simulink model "W3P3"  (R2020b)
settings: Solver=VariableStepAuto  StartTime=0.0  StopTime=10.0  RelTol=1e-3
undefined symbols (not defined in the file or in its folder): DOWN_TABLE, DOWN_TH_BP, EMAP, Iei, Kfactor, NE_VEC, speedratio, TH_VEC, Torkratio, UP_TABLE, UP_TH_BP
settings Model: Creator=saadh  LastModifiedBy=saadh

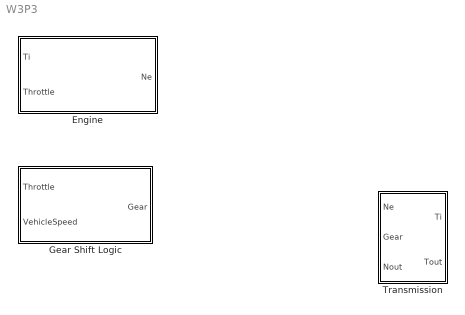
== system W3P3 ==
  Engine : Subsystem
  Gear Shift Logic : Stateflow chart  TreatAsAtomicUnit=on
  Transmission : Subsystem

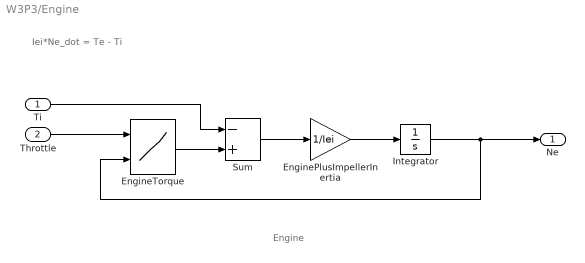
== system W3P3/Engine ==
  note: Engine
  note: Iei*Ne_dot = Te - Ti
  Ti : Inport  Unit=ft*lbf@torque
  Throttle : Inport  Port=2  Unit=%
  EnginePlusImpellerInertia : Gain  Gain=1/Iei  SaturateOnIntegerOverflow=on  OutDataTypeStr=Inherit: Same as input  ParamDataTypeStr=Inherit: Same as input
  EngineTorque : Lookup_n-D  BreakpointsForDimension1=TH_VEC  BreakpointsForDimension2=NE_VEC  Table=EMAP  InputSameDT=on
      settings: InputPortMap=u0,u1
  Integrator : Integrator  InitialCondition=1000  LimitOutput=on  UpperSaturationLimit=6000  LowerSaturationLimit=600  ZeroCross=off
  Sum : Sum  Inputs=-+  InputSameDT=on  SaturateOnIntegerOverflow=on  OutDataTypeStr=Inherit: Same as first input
  Ne : Outport  Unit=rpm  VectorParamsAs1DForOutWhenUnconnected=off
  wires:
  EngineTorque/1 -> Sum/2
  EnginePlusImpellerInertia/1 -> Integrator/1
  Integrator/1 -> Ne/1, EngineTorque/2
  Sum/1 -> EnginePlusImpellerInertia/1
  Throttle/1 -> EngineTorque/1
  Ti/1 -> Sum/1

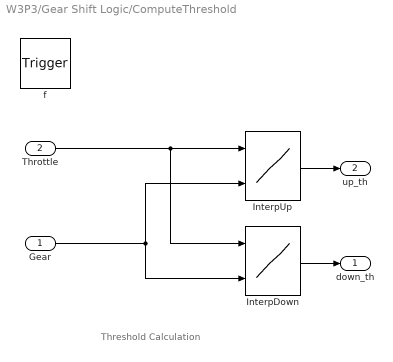
== system W3P3/Gear Shift Logic/ComputeThreshold ==
  note: Threshold Calculation
  Gear : Inport
  Throttle : Inport  Port=2
  f : TriggerPort  TriggerType=function-call  VariantControl=(inherit)
      settings: CopyFcn=Stateflow.SLINSF.SimulinkMan.removeBlockPreDeleteFcn  PreDeleteFcn=Stateflow.SLINSF.SimulinkMan.unsafePredeleteFcn
  InterpDown : Lookup_n-D  BreakpointsForDimension1=DOWN_TH_BP  BreakpointsForDimension2=[1:4]  Table=DOWN_TABLE  OutDataTypeStr=double  LockScale=on
      settings: InputPortMap=u0,u1
  InterpUp : Lookup_n-D  BreakpointsForDimension1=UP_TH_BP  BreakpointsForDimension2=[1:4]  Table=UP_TABLE  OutDataTypeStr=double  LockScale=on
      settings: InputPortMap=u0,u1
  down_th : Outport  InitialOutput=0  VectorParamsAs1DForOutWhenUnconnected=off
  up_th : Outport  Port=2  InitialOutput=0  VectorParamsAs1DForOutWhenUnconnected=off
  wires:
  Gear/1 -> InterpDown/2, InterpUp/2
  InterpUp/1 -> up_th/1
  Throttle/1 -> InterpDown/1, InterpUp/1
  InterpDown/1 -> down_th/1

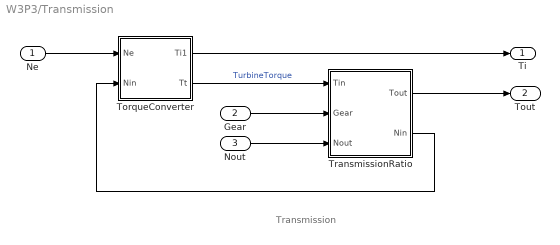
== system W3P3/Transmission ==
  note: Transmission
  Ne : Inport
  Gear : Inport  Port=2  Unit=1
  Nout : Inport  Port=3  Unit=rpm
  TorqueConverter : Subsystem
  TransmissionRatio : Subsystem
  Ti : Outport  VectorParamsAs1DForOutWhenUnconnected=off
  Tout : Outport  Port=2  Unit=ft*lbf@torque  VectorParamsAs1DForOutWhenUnconnected=off
  wires:
  Ne/1 -> TorqueConverter/1(Ne)
  TorqueConverter/2(Tt) -> TransmissionRatio/1(Tin)  "TurbineTorque"
  TransmissionRatio/1(Tout) -> Tout/1
  Gear/1 -> TransmissionRatio/2(Gear)
  TransmissionRatio/2(Nin) -> TorqueConverter/2(Nin)
  TorqueConverter/1(Ti1) -> Ti/1
  Nout/1 -> TransmissionRatio/3(Nout)

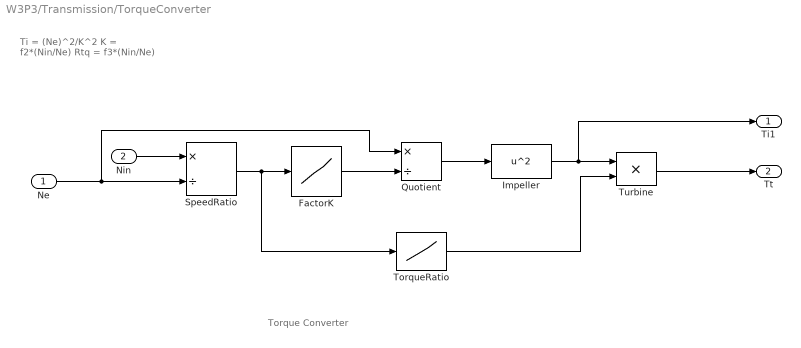
== system W3P3/Transmission/TorqueConverter ==
  note: Ti = (Ne)^2/K^2
      | K = f2*(Nin/Ne)
      | Rtq = f3*(Nin/Ne)
  note: Torque Converter
  Ne : Inport
  Nin : Inport  Port=2
  FactorK : Lookup_n-D  NumberOfTableDimensions=1  BreakpointsForDimension1=speedratio  Table=Kfactor  SaturateOnIntegerOverflow=on  InputSameDT=on
  Impeller : Fcn  Expr=u^2
  Quotient : Product  Inputs=*/  InputSameDT=on  SaturateOnIntegerOverflow=on  OutDataTypeStr=Inherit: Same as first input
  SpeedRatio : Product  Inputs=*/  InputSameDT=on  SaturateOnIntegerOverflow=on  OutDataTypeStr=Inherit: Same as first input
  TorqueRatio : Lookup_n-D  NumberOfTableDimensions=1  BreakpointsForDimension1=speedratio  Table=Torkratio  SaturateOnIntegerOverflow=on  InputSameDT=on
  Turbine : Product  InputSameDT=on  SaturateOnIntegerOverflow=on  OutDataTypeStr=Inherit: Same as first input
  Ti1 : Outport  VectorParamsAs1DForOutWhenUnconnected=off
  Tt : Outport  Port=2  VectorParamsAs1DForOutWhenUnconnected=off
  wires:
  TorqueRatio/1 -> Turbine/2
  Turbine/1 -> Tt/1
  Ne/1 -> Quotient/1, SpeedRatio/2
  Impeller/1 -> Ti1/1, Turbine/1
  Nin/1 -> SpeedRatio/1
  SpeedRatio/1 -> FactorK/1, TorqueRatio/1
  FactorK/1 -> Quotient/2
  Quotient/1 -> Impeller/1

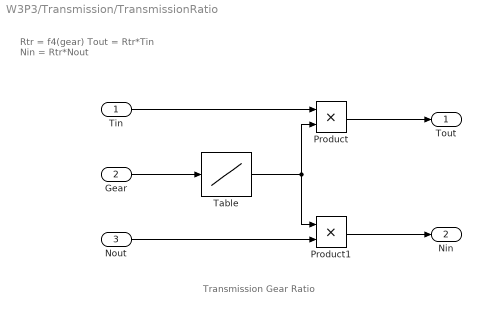
== system W3P3/Transmission/TransmissionRatio ==
  note: Rtr = f4(gear)
      | Tout = Rtr*Tin
      | Nin = Rtr*Nout
  note: Transmission Gear Ratio
  Tin : Inport  Unit=ft*lbf@torque
  Gear : Inport  Port=2  Unit=1
  Nout : Inport  Port=3  Unit=rpm
  Product : Product  InputSameDT=on  SaturateOnIntegerOverflow=on  OutDataTypeStr=Inherit: Same as first input
  Product1 : Product  InputSameDT=on  SaturateOnIntegerOverflow=on  OutDataTypeStr=Inherit: Same as first input
  Table : Lookup_n-D  NumberOfTableDimensions=1  BreakpointsForDimension1=[1 2 3 4]  Table=[2.393 1.450 1.000 0.677]  ExtrapMethod=Clip  OutDataTypeStr=double  SaturateOnIntegerOverflow=on  InputSameDT=on  LockScale=on
  Tout : Outport  Unit=ft*lbf@torque  VectorParamsAs1DForOutWhenUnconnected=off
  Nin : Outport  Port=2  Unit=rpm  VectorParamsAs1DForOutWhenUnconnected=off
  wires:
  Table/1 -> Product1/1, Product/2
  Product/1 -> Tout/1
  Nout/1 -> Product1/2
  Tin/1 -> Product/1
  Product1/1 -> Nin/1
  Gear/1 -> Table/1

== stateflow chart W3P3/Gear Shift Logic ==
  settings: updateMethod=DISCRETE  sampleTime=0.04
  state Gear_state [parallel]
    settings: executionOrder=1
    state First
      entry:
      Gear = 1;
    state Second
      entry:
      Gear = 2;
    state Third
      entry:
      Gear = 3;
    state Fourth
      entry:
      Gear = 4;
    (default) -> First
    Third -> Fourth [order 1] : UP
    Second -> Third [order 1] : UP
    First -> Second : UP
    Second -> First [order 2] : DOWN
    Third -> Second [order 2] : DOWN
    Fourth -> Third : DOWN
  state Selection_state [parallel]
    during:
    [down_th,up_th] = ComputeThreshold(Gear,Throttle)
    settings: executionOrder=2
    state Steady_state
    state Upshift
    state Downshift
    (default) -> Steady_state
    Steady_state -> Downshift [order 2] : [CheckSpeed(VehicleSpeed,up_th) == -1]
    Steady_state -> Upshift [order 1] : [CheckSpeed(VehicleSpeed,up_th) == 1]
    Downshift -> Steady_state [order 2] : [CheckSpeed(VehicleSpeed,up_th) == 1]
    Downshift -> Steady_state [order 1] : after(TWAIT,tick)
        | [VehicleSpeed <= down_th]
        | {DOWN}
    Upshift -> Steady_state [order 1] : after(TWAIT,tick)
        | [VehicleSpeed >= up_th]
        | {UP}
    Upshift -> Steady_state [order 2] : [CheckSpeed(VehicleSpeed,up_th) == -1]
  state [down_th,up_th] = ComputeThreshold(Gear,Throttle) [function]
  data: vs function_input double; threshold function_input double; speed function_output double; Gear function_input; Throttle function_input; down_th function_output; up_th function_output; Gear output fixdt(0,8,5) [1..4]; Throttle input double; VehicleSpeed input double; down_th local double; up_th local double; TWAIT parameter fixdt(0,8,6)
  events: UP local FUNCTION_CALL_EVENT; DOWN local FUNCTION_CALL_EVENT
  function speed = CheckSpeed(vs,threshold):
    | function speed = CheckSpeed(vs,threshold)
    | if(vs > threshold)
    |     speed = 1;
    | elseif(vs < threshold)
    |     speed = -1;
    | else
    |     speed = 0;
    | end
